simulink model "solving_differencial_equation"  (R2021a)
settings: Solver=VariableStepAuto  StartTime=0.0  StopTime=10.0  RelTol=1e-3
settings Model: Creator=DELL  LastModifiedBy=DELL

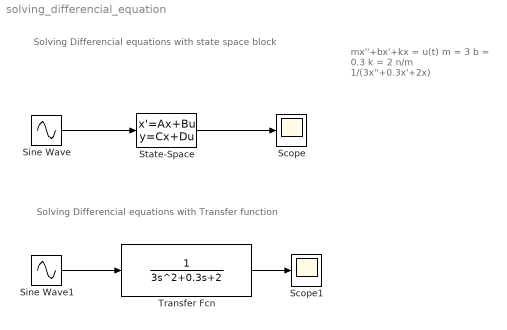
== system solving_differencial_equation ==
  note: mx''+bx'+kx = u(t)
      | m = 3
      | b = 0.3
      | k = 2 n/m
      |
      | 1/(3x''+0.3x'+2x)
  note: Solving Differencial equations with state space block
  note: Solving Differencial equations with Transfer function
  Scope : Scope
  Scope1 : Scope
  Sine Wave : Sin  SampleTime=0
  Sine Wave1 : Sin  SampleTime=0
  State-Space : StateSpace  A=[-.3/3, -2/3; 1, 0];  B=[1/3; 0];  C=[0,1];  D=0  InitialCondition=[0;1]
  Transfer Fcn : TransferFcn  Denominator="[3 0.3  2]"
  wires:
  Sine Wave/1 -> State-Space/1
  State-Space/1 -> Scope/1
  Sine Wave1/1 -> Transfer Fcn/1
  Transfer Fcn/1 -> Scope1/1
